simulink model "Pulmon"  (R2018a)
settings: Solver=VariableStepAuto  StartTime=0.0  StopTime=10.0  RelTol=1e-3
settings Model: Creator=Ruben  LastModifiedBy=Ruben

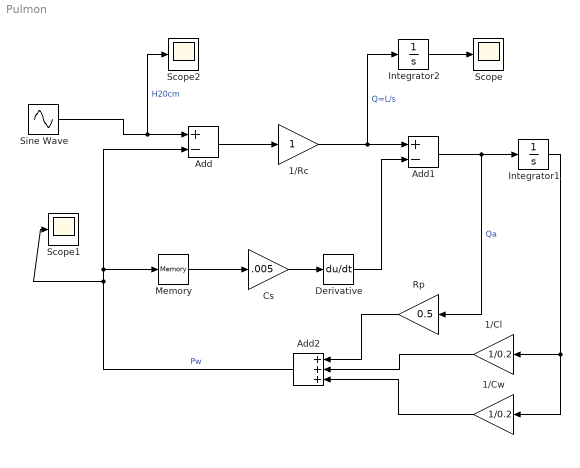
== system Pulmon ==
  1/Cl : Gain  Gain=1/0.2
  1/Cw : Gain  Gain=1/0.2
  1/Rc : Gain
  Add : Sum  Inputs=+-
  Add1 : Sum  Inputs=+-
  Add2 : Sum  Inputs=+++
  Cs : Gain  Gain=.005
  Derivative : Derivative
  Integrator1 : Integrator
  Integrator2 : Integrator
  Memory : Memory
  Rp : Gain  Gain=0.5
  Scope : Scope
  Scope1 : Scope
  Scope2 : Scope
  Sine Wave : Sin  Amplitude=2.5  Frequency=1.57  SampleTime=0
  wires:
  Memory/1 -> Cs/1
  1/Rc/1 -> Integrator2/1, Add1/1  "Q=L/s"
  Cs/1 -> Derivative/1
  Derivative/1 -> Add1/2
  Add1/1 -> Rp/1, Integrator1/1  "Qa"
  Integrator1/1 -> 1/Cw/1, 1/Cl/1
  Rp/1 -> Add2/1
  1/Cl/1 -> Add2/2
  1/Cw/1 -> Add2/3
  Add2/1 -> Scope1/1, Memory/1, Add/2  "Pw"
  Add/1 -> 1/Rc/1
  Sine Wave/1 -> Scope2/1, Add/1  "H20cm"
  Integrator2/1 -> Scope/1
